simulink library "csu_afm_aerodynamics_lib"  (R2014b)
settings: Solver=ode45  StartTime=0.0  StopTime=10.0  RelTol=1e-3
values from neighbouring files (symbols this model uses):
  AeroData =     [AeroData.mat]
  afm_cg_enable = 1    [csu_afm_aerodynamics_init.m]    (also in unit_test_aero.m = 0)
  afm_forces_enable = 1    [csu_afm_aerodynamics_init.m]
  afm_gust_direction = 0.0    (= 0)    [csu_afm_aerodynamics_init.m]
  afm_gust_length = 1.0    (= 1)    [csu_afm_aerodynamics_init.m]
  afm_gust_magnitude = 0.0    (= 0)    [csu_afm_aerodynamics_init.m]
  afm_gust_number = 1    [csu_afm_aerodynamics_init.m]
  afm_gust_start = 0.0    (= 0)    [csu_afm_aerodynamics_init.m]
  afm_moments_enable = 1    [csu_afm_aerodynamics_init.m]
  afm_winds_enable = 1    [csu_afm_aerodynamics_init.m]    (also in unit_test_aero.m = 0; unit_test_winds.m)
undefined symbols (not defined in the file or in its folder): CM
libraries: simulink_need_slupdate x49, util_common_lib x17, simulink_extras x10, simulink x7, util_quat_lib x6, util_info_lib x2, util_frame_rotation_lib x2
(part 2 of 2)

== system csu_afm_aerodynamics_lib/csu_afm_aerodynamics_mtv/COESA_1976_Atmosphere ==
  Altitude : Inport
  Alt_PreLookup : simulink_need_slupdate/PreLookup Index Search  bpData=COESA_1976.arrZ  searchMode=Binary Search  cacheBpFlag=off  outputFlag=off  IndexDataType=uint32  extrapMode=Clip to Range  rangeErrorMode=None
  Bus Creator : BusCreator  Inputs=13
  Constant1 : Constant  Value=P0
  Constant2 : Constant  Value=rho0
  Divide : Product  Inputs=*/
  Divide1 : Product  Inputs=*/
  DocBlock : simulink/Model-Wide Utilities/DocBlock  DocumentType=Text
      content=|
      | U.S. Standard Atmosphere, 1976 (COESA 1976)
      |
      | DESCRIPTION
      |    The 1976 U.S. Standard Atmosphere (COESA 1976) is an idealized,
      | steady-state representation of the earth's atmosphere from the surface
      | to 1000 km, { -5 km to 1000 km / -16,404 feet to 3,280,840 feet } as it
      | is assumed to exist in a period of moderate solar activity.
      |
      |   For the lower altitude region (-5 km to 86 km / -16404 ft to 282,152 ft),
      | simple equations can be utilized to compute the desired output values.
      | Here the gases are considered homogeneous.
      |
      |    For the upper atmospheric regions (86 km to 1000 km / 282,152 ft to
      | 3,280,840 ft), these gases undergo dissociation and diffusion.  Since the
      | gases are no longer homogeneous, more sophisticated equations are utilized
      | to correctly model values like the dominant gases' (N2, O, O2, Ar, He, H)
      | number densities.  Since integrations are used in these equations,
      | temperature and pressure computations based on these densities carry large
      | processing times.  To avoid such delays, temperature (both kinetic and
      | molecular), pressure, and air density tables have been generated at 10 m
      | (3313.6 feet) intervals using the DOS executable in Reference 2.
      |
      | NEEDED REFERENCE FILE
      |  Filename: COESA_1976.mat (Generated with 'Build_COESA_1976.m')
      |  Description: Matlab Structure Based on Data Generated by Ref 2.
      |  Form:
      |    REF_Coesa1976       {structure}             COESA 1976
      |        .AllUnits       [1x1 struct]            Units by Parameters
      |        .Description    [1x1 struct]            Description of each .arrXX
      |        .arrZ           [100501x1]  [m]         Geometric Altitude
      |        .arrT_K         [100501x1]  [deg K]     Kinetic Temperature
      |        .arrTm_K        [100501x1]  [deg K]     Molecular Temperature
      |        .arrPress       [100501x1]  [Pa]        Atmospheric Pressure
      |        .arrDensity     [100501x1]  [kg/m^3]    Atmospheric Density
      |        .arrSound       [100501x1]  [m/s]       Speed of Sound
      |        .arrmu          [100501x1]  [N-s/m^2]   Dynamic Viscosity
      |        .arreta         [100501x1]  [m^2/s]     Kinematic Viscosity
      |        .arrkt          [100501x1]  [W/(m-K)]   Coef of Thermal Conductivity
      |
      | SOURCES
      |   Reference 1:
      |    COESA (Committee on Extension to the Standard Atmosphere), U.S.
      |    Standard Atmosphere 1976, U.S. Government Printing Office,
      |    Washington, DC, October 1976.
      |
      |   Reference 2:
      |    "U.S. Standard Atmopsphere 1976"
      |    Online References found through NASA Goddard Space Flight Center
      |
      |    Main Description:
      |      http://nssdc.gsfc.nasa.gov/space/model/atmos/us_standard.html
      |    Turbo Pascal Source Code
      |      http://www.sworld.com.au/steven/space/atmosphere/
      |      Note: This website contains corrections to Reference 1
  Geopotential_Height_m : Subsystem
  Table_Density : simulink_need_slupdate/Interpolation (n-D) using PreLookup  numDimsPopupSelect=1  explicitNumDims=2  table=COESA_1976.arrDensity  interpMethod=Linear  extrapMethod=None - Clip  rangeErrorMode=None  NumSelectionDims=0
  Table_DynamicViscosity : simulink_need_slupdate/Interpolation (n-D) using PreLookup  numDimsPopupSelect=1  explicitNumDims=2  table=COESA_1976.arrmu  interpMethod=Linear  extrapMethod=None - Clip  rangeErrorMode=None  NumSelectionDims=0
  Table_KinematicViscosity : simulink_need_slupdate/Interpolation (n-D) using PreLookup  numDimsPopupSelect=1  explicitNumDims=2  table=COESA_1976.arreta  interpMethod=Linear  extrapMethod=None - Clip  rangeErrorMode=None  NumSelectionDims=0
  Table_Kinetic_Temp : simulink_need_slupdate/Interpolation (n-D) using PreLookup  numDimsPopupSelect=1  explicitNumDims=2  table=COESA_1976.arrT_K  interpMethod=Linear  extrapMethod=None - Clip  rangeErrorMode=None  NumSelectionDims=0
  Table_MeanFreePath : simulink_need_slupdate/Interpolation (n-D) using PreLookup  numDimsPopupSelect=1  explicitNumDims=2  table=COESA_1976.arrL  interpMethod=Linear  extrapMethod=None - Clip  rangeErrorMode=None  NumSelectionDims=0
  Table_Molecular_Temp : simulink_need_slupdate/Interpolation (n-D) using PreLookup  numDimsPopupSelect=1  explicitNumDims=2  table=COESA_1976.arrTm_K  interpMethod=Linear  extrapMethod=None - Clip  rangeErrorMode=None  NumSelectionDims=0
  Table_Pressure : simulink_need_slupdate/Interpolation (n-D) using PreLookup  numDimsPopupSelect=1  explicitNumDims=2  table=COESA_1976.arrPress  interpMethod=Linear  extrapMethod=None - Clip  rangeErrorMode=None  NumSelectionDims=0
  Table_SpeedofSound : simulink_need_slupdate/Interpolation (n-D) using PreLookup  numDimsPopupSelect=1  explicitNumDims=2  table=COESA_1976.arrSound  interpMethod=Linear  extrapMethod=None - Clip  rangeErrorMode=None  NumSelectionDims=0
  Table_ThermalConductivity : simulink_need_slupdate/Interpolation (n-D) using PreLookup  numDimsPopupSelect=1  explicitNumDims=2  table=COESA_1976.arrkt  interpMethod=Linear  extrapMethod=None - Clip  rangeErrorMode=None  NumSelectionDims=0
  AtmosphereBus : Outport
  wires:
  Alt_PreLookup/1 -> Table_MeanFreePath/1, Table_ThermalConductivity/1, Table_KinematicViscosity/1, Table_DynamicViscosity/1, Table_SpeedofSound/1, Table_Density/1, Table_Pressure/1, Table_Molecular_Temp/1, Table_Kinetic_Temp/1
  Table_ThermalConductivity/1 -> Bus Creator/12  "kt"
  Table_KinematicViscosity/1 -> Bus Creator/11  "KinematicViscosity"
  Table_SpeedofSound/1 -> Bus Creator/9  "Sound"
  Table_MeanFreePath/1 -> Bus Creator/13  "MeanFreePath"
  Bus Creator/1 -> AtmosphereBus/1
  Table_DynamicViscosity/1 -> Bus Creator/10  "DynamicViscosity"
  Divide1/1 -> Bus Creator/8  "RhoRho0"
  Constant2/1 -> Divide1/2
  Constant1/1 -> Divide/2
  Divide/1 -> Bus Creator/6  "PP0"
  Geopotential_Height_m/1(H_m) -> Bus Creator/2  "GeopotentialAlt"
  Altitude/1 -> Alt_PreLookup/1, Geopotential_Height_m/1(Z_m), Bus Creator/1  "GeometricAlt"
  Table_Density/1 -> Divide1/1, Bus Creator/7  "Density"
  Table_Pressure/1 -> Divide/1, Bus Creator/5  "Pressure"
  Table_Molecular_Temp/1 -> Bus Creator/4  "Temp_Molecular"
  Table_Kinetic_Temp/1 -> Bus Creator/3  "Temp_Kinetic"

== system csu_afm_aerodynamics_lib/csu_afm_aerodynamics_mtv/CheckForZero ==
  In : Inport
  Constant : Constant  Value=0
  Gain : Gain  Gain=eps
  Logical Operator1 : Logic  Operator=NOT  AllPortsSameDT=off  OutDataTypeStr=float('double')
  Product : Product  RndMeth=Zero
  Relational Operator : RelationalOperator  Operator===  OutDataTypeStr=float('double')
  Sum : Sum  Inputs=|++
  Out : Outport
  wires:
  Constant/1 -> Relational Operator/2
  Sum/1 -> Out/1
  Product/1 -> Sum/1
  Logical Operator1/1 -> Product/2
  Gain/1 -> Sum/2
  Relational Operator/1 -> Logical Operator1/1, Gain/1
  In/1 -> Relational Operator/1, Product/1

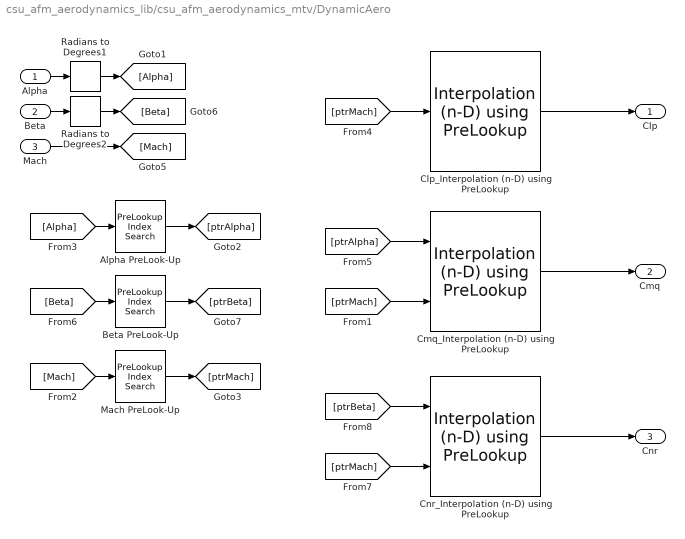
== system csu_afm_aerodynamics_lib/csu_afm_aerodynamics_mtv/DynamicAero ==
  Alpha : Inport
  Beta : Inport  Port=2
  Mach : Inport  Port=3
  Alpha PreLook-Up : simulink_need_slupdate/PreLookup Index Search  bpData=AeroData.Dynamic.Alpha  searchMode=Binary Search  cacheBpFlag=on  outputFlag=off  IndexDataType=uint32  extrapMode=Clip to Range  rangeErrorMode=None
  Beta PreLook-Up : simulink_need_slupdate/PreLookup Index Search  bpData=AeroData.Dynamic.Beta  searchMode=Binary Search  cacheBpFlag=on  outputFlag=off  IndexDataType=uint32  extrapMode=Clip to Range  rangeErrorMode=None
  Clp_Interpolation (n-D) using PreLookup : simulink_need_slupdate/Interpolation (n-D) using PreLookup  numDimsPopupSelect=1  explicitNumDims=2  table=AeroData.Dynamic.Clp  interpMethod=Linear  extrapMethod=None - Clip  rangeErrorMode=None  NumSelectionDims=0
  Cmq_Interpolation (n-D) using PreLookup : simulink_need_slupdate/Interpolation (n-D) using PreLookup  numDimsPopupSelect=2  explicitNumDims=2  table=AeroData.Dynamic.Cmq  interpMethod=Linear  extrapMethod=None - Clip  rangeErrorMode=None  NumSelectionDims=0
  Cnr_Interpolation (n-D) using PreLookup : simulink_need_slupdate/Interpolation (n-D) using PreLookup  numDimsPopupSelect=2  explicitNumDims=2  table=AeroData.Dynamic.Cnr  interpMethod=Linear  extrapMethod=None - Clip  rangeErrorMode=None  NumSelectionDims=0
  Mach PreLook-Up : simulink_need_slupdate/PreLookup Index Search  bpData=AeroData.Dynamic.Mach  searchMode=Binary Search  cacheBpFlag=on  outputFlag=off  IndexDataType=uint32  extrapMode=Clip to Range  rangeErrorMode=None
  Radians to Degrees1 : simulink_extras/Transformations/Radians to Degrees
  Radians to Degrees2 : simulink_extras/Transformations/Radians to Degrees
  Clp : Outport  PortDimensions=1  InitialOutput=CM.Aero.DynamicData.CM_only.Clp
  Cmq : Outport  Port=2  PortDimensions=1  InitialOutput=0
  Cnr : Outport  Port=3  PortDimensions=1  InitialOutput=0
  wires:
  [ptrMach] -> Clp_Interpolation (n-D) using PreLookup/1
  Clp_Interpolation (n-D) using PreLookup/1 -> Clp/1
  Mach/1 -> [Mach]
  [ptrAlpha] -> Cmq_Interpolation (n-D) using PreLookup/1
  [ptrMach] -> Cmq_Interpolation (n-D) using PreLookup/2
  [ptrBeta] -> Cnr_Interpolation (n-D) using PreLookup/1
  [ptrMach] -> Cnr_Interpolation (n-D) using PreLookup/2
  Alpha PreLook-Up/1 -> [ptrAlpha]
  Mach PreLook-Up/1 -> [ptrMach]
  [Alpha] -> Alpha PreLook-Up/1
  [Mach] -> Mach PreLook-Up/1
  Beta PreLook-Up/1 -> [ptrBeta]
  [Beta] -> Beta PreLook-Up/1
  Cmq_Interpolation (n-D) using PreLookup/1 -> Cmq/1
  Cnr_Interpolation (n-D) using PreLookup/1 -> Cnr/1
  Radians to Degrees1/1 -> [Alpha]
  Radians to Degrees2/1 -> [Beta]
  Beta/1 -> Radians to Degrees2/1
  Alpha/1 -> Radians to Degrees1/1

== system csu_afm_aerodynamics_lib/csu_afm_aerodynamics_mtv/EarthRotMatrix ==
  Constant{1..7} (7 alike) : Constant  Value=0
  EarthRate : Constant  Value=7.2921151467e-5
  Gain1 : Gain  Gain=-1  SaturateOnIntegerOverflow=on  OutDataTypeStr=Inherit: Same as input  ParamDataTypeStr=Inherit: Same as input
  Matrix Concatenation : Concatenate  NumInputs=3  Mode=Multidimensional array  ConcatenateDimension=2
  Mux : Mux  Inputs=3
  Mux1 : Mux  Inputs=3
  Mux2 : Mux  Inputs=3
  EarthRotationMatrix : Outport
  wires:
  Mux2/1 -> Matrix Concatenation/3
  Matrix Concatenation/1 -> EarthRotationMatrix/1
  EarthRate/1 -> [omegaE]
  [omegaE] -> Mux/2
  Constant5/1 -> Mux/1
  Constant6/1 -> Mux/3
  Constant4/1 -> Mux1/2
  Constant7/1 -> Mux2/3
  Constant3/1 -> Mux2/2
  Constant1/1 -> Mux2/1
  Constant2/1 -> Mux1/3
  Gain1/1 -> Mux1/1
  Mux1/1 -> Matrix Concatenation/2
  Mux/1 -> Matrix Concatenation/1
  [omegaE] -> Gain1/1

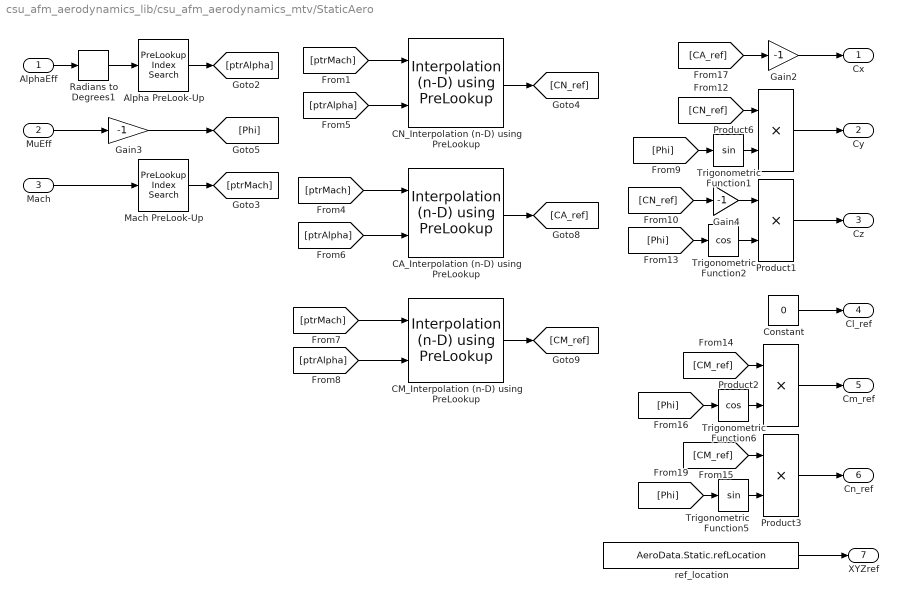
== system csu_afm_aerodynamics_lib/csu_afm_aerodynamics_mtv/StaticAero ==
  AlphaEff : Inport
  MuEff : Inport  Port=2
  Mach : Inport  Port=3
  Alpha PreLook-Up : simulink_need_slupdate/PreLookup Index Search  bpData=AeroData.Static.Alpha  searchMode=Binary Search  cacheBpFlag=on  outputFlag=off  IndexDataType=uint32  extrapMode=Clip to Range  rangeErrorMode=None
  CA_Interpolation (n-D) using PreLookup : simulink_need_slupdate/Interpolation (n-D) using PreLookup  numDimsPopupSelect=2  explicitNumDims=2  table=AeroData.Static.CA  interpMethod=Linear  extrapMethod=None - Clip  rangeErrorMode=None  NumSelectionDims=0
  CM_Interpolation (n-D) using PreLookup : simulink_need_slupdate/Interpolation (n-D) using PreLookup  numDimsPopupSelect=2  explicitNumDims=2  table=AeroData.Static.CM  interpMethod=Linear  extrapMethod=None - Clip  rangeErrorMode=None  NumSelectionDims=0
  CN_Interpolation (n-D) using PreLookup : simulink_need_slupdate/Interpolation (n-D) using PreLookup  numDimsPopupSelect=2  explicitNumDims=2  table=AeroData.Static.CN  interpMethod=Linear  extrapMethod=None - Clip  rangeErrorMode=None  NumSelectionDims=0
  Constant : Constant  Value=0
  Gain2 : Gain  Gain=-1
  Gain3 : Gain  Gain=-1
  Gain4 : Gain  Gain=-1
  Mach PreLook-Up : simulink_need_slupdate/PreLookup Index Search  bpData=AeroData.Static.Mach  searchMode=Binary Search  cacheBpFlag=on  outputFlag=off  IndexDataType=uint32  extrapMode=Clip to Range  rangeErrorMode=None
  Product{1..3,6} (4 alike) : Product  SaturateOnIntegerOverflow=on  OutDataTypeStr=Inherit: Same as first input
  Radians to Degrees1 : simulink_extras/Transformations/Radians to Degrees
  Trigonometric Function1 : Trigonometry
  Trigonometric Function2 : Trigonometry  Operator=cos
  Trigonometric Function5 : Trigonometry
  Trigonometric Function6 : Trigonometry  Operator=cos
  ref_location : Constant  Value=AeroData.Static.refLocation
  Cx : Outport
  Cy : Outport  Port=2
  Cz : Outport  Port=3
  Cl_ref : Outport  Port=4
  Cm_ref : Outport  Port=5
  Cn_ref : Outport  Port=6
  XYZref : Outport  Port=7  InitialOutput=[0 0 0]
  wires:
  ref_location/1 -> XYZref/1
  Radians to Degrees1/1 -> Alpha PreLook-Up/1
  Gain4/1 -> Product1/1
  Gain3/1 -> [Phi]
  Product3/1 -> Cn_ref/1
  Product2/1 -> Cm_ref/1
  [CM_ref] -> Product2/1
  Trigonometric Function5/1 -> Product3/2
  [Phi] -> Trigonometric Function5/1
  [CM_ref] -> Product3/1
  Trigonometric Function6/1 -> Product2/2
  [Phi] -> Trigonometric Function6/1
  Product1/1 -> Cz/1
  [CN_ref] -> Gain4/1
  Trigonometric Function1/1 -> Product6/2
  [Phi] -> Trigonometric Function1/1
  [CN_ref] -> Product6/1
  Constant/1 -> Cl_ref/1
  Trigonometric Function2/1 -> Product1/2
  [Phi] -> Trigonometric Function2/1
  Product6/1 -> Cy/1
  Gain2/1 -> Cx/1
  Mach/1 -> Mach PreLook-Up/1
  [ptrAlpha] -> CM_Interpolation (n-D) using PreLookup/2
  [ptrMach] -> CM_Interpolation (n-D) using PreLookup/1
  [ptrAlpha] -> CA_Interpolation (n-D) using PreLookup/2
  [ptrMach] -> CA_Interpolation (n-D) using PreLookup/1
  [ptrAlpha] -> CN_Interpolation (n-D) using PreLookup/2
  [ptrMach] -> CN_Interpolation (n-D) using PreLookup/1
  [CA_ref] -> Gain2/1
  CM_Interpolation (n-D) using PreLookup/1 -> [CM_ref]
  CA_Interpolation (n-D) using PreLookup/1 -> [CA_ref]
  CN_Interpolation (n-D) using PreLookup/1 -> [CN_ref]
  MuEff/1 -> Gain3/1
  AlphaEff/1 -> Radians to Degrees1/1
  Mach PreLook-Up/1 -> [ptrMach]
  Alpha PreLook-Up/1 -> [ptrAlpha]

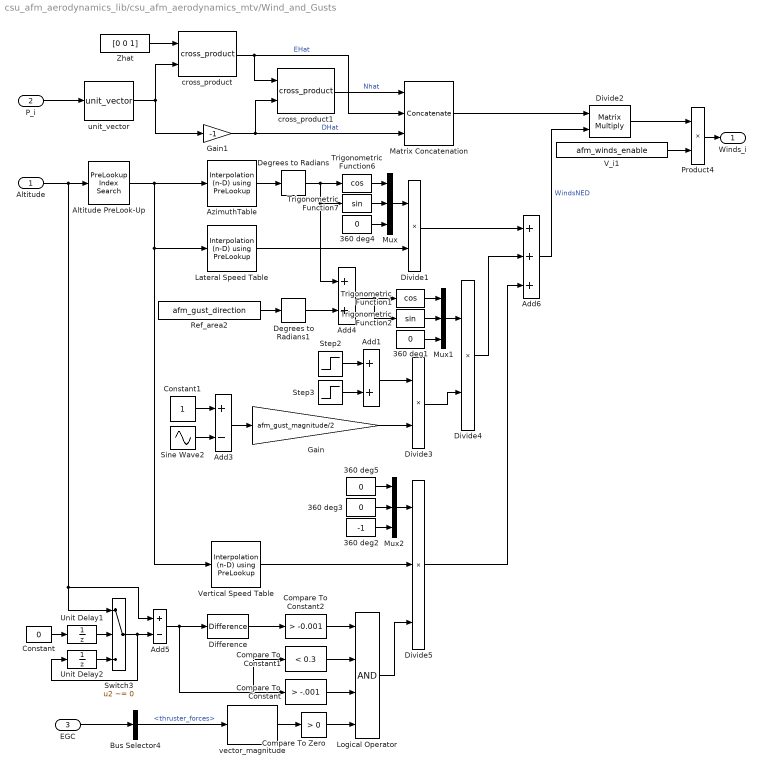
== system csu_afm_aerodynamics_lib/csu_afm_aerodynamics_mtv/Wind_and_Gusts ==
  Altitude : Inport  PortDimensions=1
  P_i : Inport  Port=2  PortDimensions=3
  EGC : Inport  Port=3
  360 deg{1,3..5} (4 alike) : Constant  Value=0
  360 deg2 : Constant  Value=-1
  Add1 : Sum
  Add3 : Sum  Inputs=+-
  Add4 : Sum
  Add5 : Sum  Inputs=+-
  Add6 : Sum  Inputs=+++
  Altitude PreLook-Up : simulink_need_slupdate/PreLookup Index Search  bpData=Winds.Altitude  searchMode=Binary Search  cacheBpFlag=on  outputFlag=off  IndexDataType=uint32  extrapMode=Clip to Range  rangeErrorMode=None
  AzimuthTable : simulink_need_slupdate/Interpolation (n-D) using PreLookup  numDimsPopupSelect=1  explicitNumDims=2  table=Winds.Azimuth  interpMethod=Linear  extrapMethod=None - Clip  rangeErrorMode=None  NumSelectionDims=0
  Bus Selector4 : BusSelector  OutputSignals=thruster_forces
  Compare To Constant : simulink/Logic and Bit Operations/Compare To Constant  relop=>  const=-.001  OutDataTypeStr=boolean
  Compare To Constant1 : simulink/Logic and Bit Operations/Compare To Constant  relop=<  const=0.3  OutDataTypeStr=boolean
  Compare To Constant2 : simulink/Logic and Bit Operations/Compare To Constant  relop=>  const=-0.001  OutDataTypeStr=boolean
  Compare To Zero : simulink/Logic and Bit Operations/Compare To Zero  relop=>  OutDataTypeStr=boolean
  Constant : Constant  Value=0
  Constant1 : Constant
  Degrees to Radians : simulink_extras/Transformations/Degrees to Radians
  Degrees to Radians1 : simulink_extras/Transformations/Degrees to Radians
  Difference : simulink/Discrete/Difference  ICPrevInput=0.0  InputProcessing=Inherited  OutMin=[]  OutMax=[]  OutDataType=fixdt(1, 16)  OutScaling=2^-10  DoSatur=off
  Divide1 : Product  Inputs=**
  Divide2 : Product  Inputs=**  Multiplication=Matrix(*)
  Divide3 : Product  Inputs=**
  Divide4 : Product  Inputs=**
  Divide5 : Product  Inputs=***
  Gain : Gain  Gain=afm_gust_magnitude/2
  Gain1 : Gain  Gain=-1
  Lateral Speed Table : simulink_need_slupdate/Interpolation (n-D) using PreLookup  numDimsPopupSelect=1  explicitNumDims=2  table=Winds.Speed.Lateral  interpMethod=Linear  extrapMethod=None - Clip  rangeErrorMode=None  NumSelectionDims=0
  Logical Operator : Logic  Inputs=4  AllPortsSameDT=off  OutDataTypeStr=boolean
  Matrix Concatenation : Concatenate  NumInputs=3  Mode=Multidimensional array  ConcatenateDimension=2
  Mux : Mux  Inputs=3
  Mux1 : Mux  Inputs=3
  Mux2 : Mux  Inputs=3
  Product4 : Product  RndMeth=Zero
  Ref_area2 : Constant  Value=afm_gust_direction
  Sine Wave2 : Sin  Frequency=2*pi/afm_gust_length*afm_gust_number  Phase=pi/2-2*pi/afm_gust_length*afm_gust_number*afm_gust_start  SampleTime=.01  VectorParams1D=off
  Step2 : Step  Time=afm_gust_start  SampleTime=.01
  Step3 : Step  Time=afm_gust_start+afm_gust_length  After=-1  SampleTime=.01
  Switch3 : Switch  Criteria=u2 ~= 0  OutDataTypeStr=double
  Trigonometric Function1 : Trigonometry  Operator=cos
  Trigonometric Function2 : Trigonometry
  Trigonometric Function6 : Trigonometry  Operator=cos
  Trigonometric Function7 : Trigonometry
  Unit Delay1 : UnitDelay  InitialCondition=1  SampleTime=-1
  Unit Delay2 : UnitDelay  SampleTime=-1
  V_i1 : Constant  Value=afm_winds_enable  VectorParams1D=off
  Vertical Speed Table : simulink_need_slupdate/Interpolation (n-D) using PreLookup  numDimsPopupSelect=1  explicitNumDims=2  table=Winds.Speed.Vertical  interpMethod=Linear  extrapMethod=None - Clip  rangeErrorMode=None  NumSelectionDims=0
  Zhat : Constant  Value=[0 0 1]
  cross_product : util_common_lib/cross_product  SystemSampleTime=-1
  cross_product1 : util_common_lib/cross_product  SystemSampleTime=-1
  unit_vector : util_common_lib/unit_vector  SystemSampleTime=-1
  vector_magnitude : util_common_lib/vector_magnitude  SystemSampleTime=-1
  Winds_i : Outport  PortDimensions=3
  wires:
  Divide4/1 -> Add6/2
  Divide1/1 -> Add6/1
  360 deg1/1 -> Mux1/3
  Degrees to Radians1/1 -> Add4/2
  Ref_area2/1 -> Degrees to Radians1/1
  Add4/1 -> Trigonometric Function1/1, Trigonometric Function2/1
  Mux1/1 -> Divide4/1
  Trigonometric Function2/1 -> Mux1/2
  Trigonometric Function1/1 -> Mux1/1
  Sine Wave2/1 -> Add3/2
  Add3/1 -> Gain/1
  Constant1/1 -> Add3/1
  Add6/1 -> Divide2/2  "WindsNED"
  Divide3/1 -> Divide4/2
  Add1/1 -> Divide3/1
  Step3/1 -> Add1/2
  Step2/1 -> Add1/1
  Gain/1 -> Divide3/2
  Divide2/1 -> Product4/1
  V_i1/1 -> Product4/2
  AzimuthTable/1 -> Degrees to Radians/1
  P_i/1 -> unit_vector/1
  Zhat/1 -> cross_product/1
  unit_vector/1 -> cross_product/2, Gain1/1
  Degrees to Radians/1 -> Trigonometric Function6/1, Add4/1, Trigonometric Function7/1
  Product4/1 -> Winds_i/1
  Matrix Concatenation/1 -> Divide2/1
  cross_product1/1 -> Matrix Concatenation/1  "Nhat"
  cross_product/1 -> cross_product1/1, Matrix Concatenation/2  "EHat"
  Gain1/1 -> cross_product1/2, Matrix Concatenation/3  "DHat"
  Lateral Speed Table/1 -> Divide1/2
  Mux/1 -> Divide1/1
  360 deg4/1 -> Mux/3
  Trigonometric Function7/1 -> Mux/2
  Trigonometric Function6/1 -> Mux/1
  360 deg5/1 -> Mux2/1
  Difference/1 -> Compare To Constant2/1
  Compare To Constant2/1 -> Logical Operator/1
  Compare To Constant1/1 -> Logical Operator/2
  Add5/1 -> Compare To Constant/1, Compare To Constant1/1, Difference/1
  Switch3/1 -> Unit Delay2/1, Add5/2
  Unit Delay1/1 -> Switch3/2
  Constant/1 -> Unit Delay1/1
  Unit Delay2/1 -> Switch3/3
  Compare To Constant/1 -> Logical Operator/3
  Compare To Zero/1 -> Logical Operator/4
  Logical Operator/1 -> Divide5/3
  Vertical Speed Table/1 -> Divide5/2
  Bus Selector4/1 -> vector_magnitude/1  "<thruster_forces>"
  EGC/1 -> Bus Selector4/1
  vector_magnitude/1 -> Compare To Zero/1
  360 deg3/1 -> Mux2/2
  Mux2/1 -> Divide5/1
  360 deg2/1 -> Mux2/3
  Altitude/1 -> Add5/1, Switch3/1, Altitude PreLook-Up/1
  Altitude PreLook-Up/1 -> AzimuthTable/1, Lateral Speed Table/1, Vertical Speed Table/1
  Divide5/1 -> Add6/3

== system csu_afm_aerodynamics_lib/csu_afm_aerodynamics/COESA_1976_Atmosphere/Geopotential_Height_m ==
  Z_m : Inport
  Add : Sum
  Divide : Product  Inputs=*/
  Earth_Radius_m : Constant  Value=r0
  Product : Product  RndMeth=Zero
  H_m : Outport
  wires:
  Z_m/1 -> Add/2, Product/1
  Divide/1 -> H_m/1
  Add/1 -> Divide/2
  Product/1 -> Divide/1
  Earth_Radius_m/1 -> Add/1, Product/2

== system csu_afm_aerodynamics_lib/csu_afm_aerodynamics_mtv/COESA_1976_Atmosphere/Geopotential_Height_m ==
  Z_m : Inport
  Add : Sum
  Divide : Product  Inputs=*/
  Earth_Radius_m : Constant  Value=r0
  Product : Product  RndMeth=Zero
  H_m : Outport
  wires:
  Earth_Radius_m/1 -> Product/2, Add/1
  Product/1 -> Divide/1
  Add/1 -> Divide/2
  Divide/1 -> H_m/1
  Z_m/1 -> Product/1, Add/2
